simulink model "sistema_LTI"  (R2016b)
settings: Solver=VariableStepAuto  StartTime=0.0  StopTime=10.0  RelTol=1e-3
values from neighbouring files (symbols this model uses):
  Beq = bm+(bl)/r^2    (= 1.5e-05)    [c4ModeloCompleto_var.m]
  Jeq = Jm+(Jl/r^2)    (= 5.65099476805e-06)    [c4ModeloCompleto_var.m]
  lambda_m = 0.01546    [c4ModeloCompleto.m]    (also in c4ModeloCompleto_var.m)
  Lq = 5.8    [c4ModeloCompleto.m]    (also in c4ModeloCompleto_var.m = 0.0058)
  Pp = 3    [c4ModeloCompleto.m]    (also in c4ModeloCompleto_var.m)
  r = 314.3008    [c4ModeloCompleto.m]    (also in c4ModeloCompleto_var.m)
  Rs = 1.02    [c4ModeloCompleto_var.m]
settings Model: Creator=agustin  LastModifiedBy=agustin

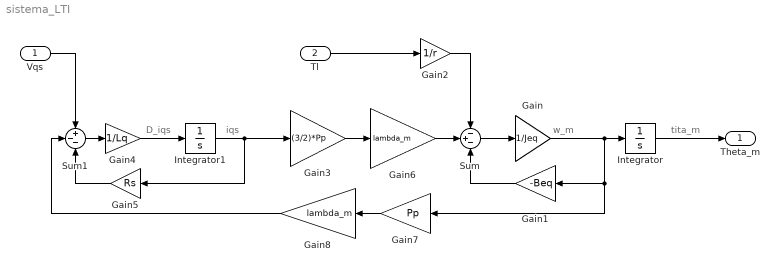
== system sistema_LTI ==
  note: tita_m
  note: w_m
  note: iqs
  note: D_iqs
  Vqs : Inport
  Tl : Inport  Port=2
  Gain : Gain  Gain=1/Jeq
  Gain1 : Gain  Gain=-Beq
  Gain2 : Gain  Gain=1/r
  Gain3 : Gain  Gain=(3/2)*Pp
  Gain4 : Gain  Gain=1/Lq
  Gain5 : Gain  Gain=Rs
  Gain6 : Gain  Gain=lambda_m
  Gain7 : Gain  Gain=Pp
  Gain8 : Gain  Gain=lambda_m
  Integrator : Integrator
  Integrator1 : Integrator
  Sum : Sum  Inputs=-+-
  Sum1 : Sum  Inputs=+--
  Theta_m : Outport
  wires:
  Gain/1 -> Gain7/1, Gain1/1, Integrator/1
  Sum/1 -> Gain/1
  Gain1/1 -> Sum/3
  Tl/1 -> Gain2/1
  Gain2/1 -> Sum/1
  Gain4/1 -> Integrator1/1
  Sum1/1 -> Gain4/1
  Integrator1/1 -> Gain5/1, Gain3/1
  Gain5/1 -> Sum1/3
  Vqs/1 -> Sum1/1
  Integrator/1 -> Theta_m/1
  Gain7/1 -> Gain8/1
  Gain3/1 -> Gain6/1
  Gain6/1 -> Sum/2
  Gain8/1 -> Sum1/2
